simulink model "Receiver"  (R2015a)
settings: Solver=ode45  StartTime=0.0  StopTime=10.0  RelTol=1e-3
libraries: xpcutilitieslib x1, xpciplib x1, xpcrtudplib x1, slrtlib x1
settings Model: xpc_rtwmakecfg_data=_xpcetherlib__xpcether8255xlib__xpcetherGbElib__xpcnblib_  Creator=Dominik  LastModifiedBy=Dominik

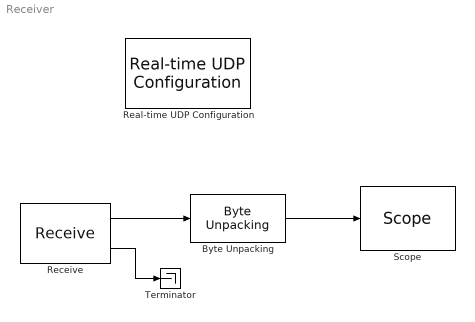
== system Receiver ==
  "Byte Unpacking " : xpcutilitieslib/Byte Unpacking   MaskUnpackedDataTypes={'double'}  MaskUnpackedDataSizes={[2]}  MaskAlignment=1
  "Real-time UDP Configuration " : xpciplib/Real-time UDP  Configuration   ID=1  IpAddress=30.30.30.2  SubnetMask=255.255.255.0  Gateway=0.0.0.0  EthDrv=Intel Gigabit  PciBus=5  PciSlot=0  udpID=0
  "Receive " : xpcrtudplib/Receive   ID=1  Receive1=30.30.30.1  Receive2=25000  Receive3=16  Receive4=-1  udpID=0
  "Scope " : slrtlib/Displays and Logging/Scope   scopeno=1  scopetype=Target  autostart=on  viewmode=Graphical redraw  formatstr='%15.6f'  grid=on  ylimits=[0,0]  nosamples=250  noprepostsamples=0  interleave=1  triggermode=FreeRun  triggersignal=1  trigsignalfromport=off  triggerlevel=0.0  triggerslope=Either  triggerscope=1  triggersample=0  filename=data.dat  mode=Lazy  writesize=512  autorestart=off  dynamicfilemode=off  maxwritefilesize=512*1024^2
  Terminator : Terminator
  wires:
  "Receive "/1 -> "Byte Unpacking "/1
  "Receive "/2 -> Terminator/1
  "Byte Unpacking "/1 -> "Scope "/1
